simulink model "Assignment3"  (R2022a)
settings: Solver=VariableStepAuto  StartTime=0.0  StopTime=10.0  RelTol=1e-3
settings Model: Creator=qiuhb  LastModifiedBy=qiuhb

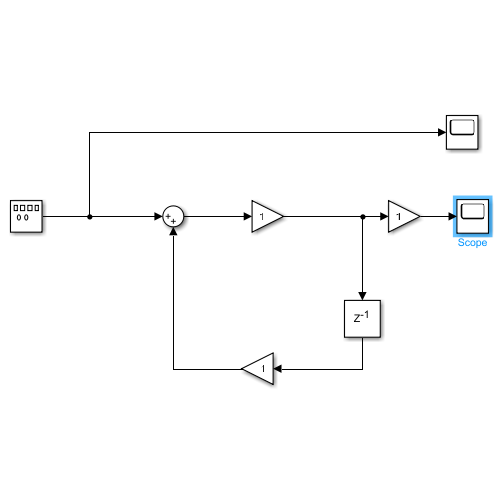
[thumbnail: Simulink's stored preview of the top-level diagram]
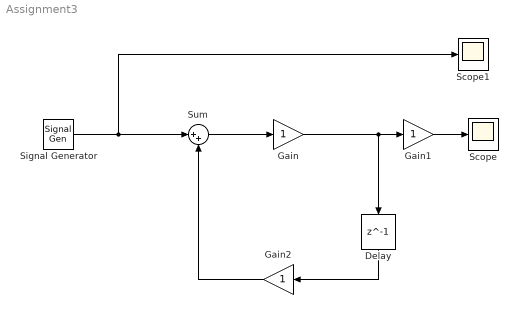
== system Assignment3 ==
  Delay : Delay  DelayLength=1  InitialCondition=0
  Gain : Gain
  Gain1 : Gain
  Gain2 : Gain
  Scope : Scope
  Scope1 : Scope
  Signal Generator : SignalGenerator  Units=rad/sec
  Sum : Sum  Inputs=|++
  wires:
  Gain/1 -> Gain1/1, Delay/1
  Sum/1 -> Gain/1
  Gain2/1 -> Sum/2
  Signal Generator/1 -> Scope1/1, Sum/1
  Gain1/1 -> Scope/1
  Delay/1 -> Gain2/1
